simulink model "switching_controller_parallel_after_retraining"  (R2020a)
settings: Solver=FixedStepAuto  StartTime=0.0  StopTime=simulation.time_window  FixedStep=simulation.time_step  MaxStep=.2  RelTol=1e-3
model workspace (MAT data in the model file):
  PID_TRESH = 0.3
undefined symbols (not defined in the file): DiscIntNeverNeededParam
libraries: neural x72, simulink x1
(part 2 of 3)

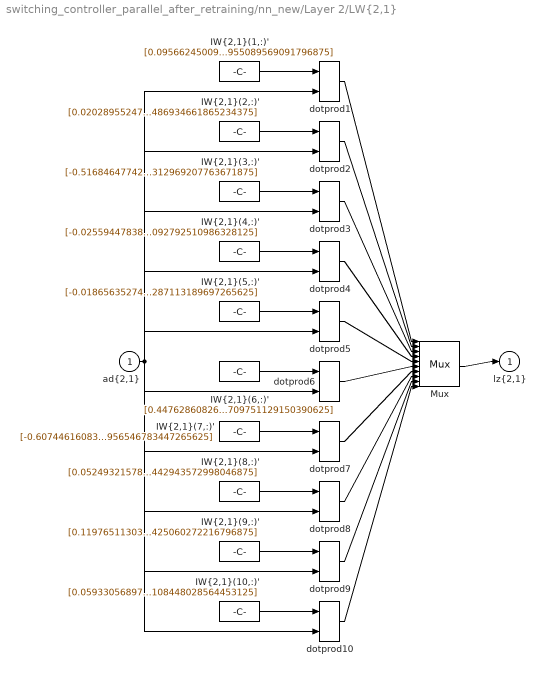
== system switching_controller_parallel_after_retraining/nn_new/Layer 2/LW{2,1} ==
  "ad{2,1}" : Inport  PortDimensions=20
      mask Display: e = 0.06;c1 = [120 230 180]/255;c2 = ([120 230 180]+0)/(256+128);c3 = ([120 230 180]+128)/(256+128);patch([0 1 1 0],[0 0 1 1],c1);patch([0 1 1 1-e 1-e 0+e],[0 0 1 1-e 0+e 0+e],c2);patch([0 0 1 1-e 0+e 0+e],[0 1 1 1-e 1-e 0+e],c3);plot([0 1 1 0 0],[0 0 1 1 0]);
  "IW{2,1}(1,:)'" : Constant  Value=[0.095662450092162620851610199679271318018436431884765625;-0.57681603256735758389339707719045691192150115966796875;0.7629740687628425721555913696647621691226959228515625;0.4894431043993183738649577207979746162891387939453125;0.044507659808209469598505592102810624055564403533935546875;0.61157764582548324039379394889692775905132293701171875;-0.322091177630037084345104858584818430244922637939453125;0.70740757035732826363272351954947225749492645263671875;-0.03743755377230949255018543908590800128877162933349609375;0.6222453992016114820984284961014054715633392333984375;0.307063272338365111924218808781006373465061187744140625;-0.2787568726492377635395314428023993968963623046875;0.059040537912539138576395458812839933671057224273681640625;-0.119200421424518143709292417042888700962066650390625;-0.151215357399669958482490983442403376102447509765625;0.33914961325253145663083387262304313480854034423828125;0.441032178568772248450358119953307323157787322998046875;-0.75715377678111384085468671401031315326690673828125;-0.2200805339957083994750774991189246065914630889892578125;0.54986307386627675253265579158323816955089569091796875]
      mask Display: e = 0.06;c1 = [120 150 230]/255;c2 = ([120 150 230]+0)/383;c3 = ([120 150 230]+128)/383;patch([0 1 1 0],[0 0 1 1],c1);patch([0 1 1 1-e 1-e 0+e],[0 0 1 1-e 0+e 0+e],c2);patch([0 0 1 1-e 0+e 0+e],[0 1 1 1-e 1-e 0+e],c3);plot([0 1 1 0 0],[0 0 1 1 0]);disp('weights');
  "IW{2,1}(10,:)'" : Constant  Value=[0.05933056897562051512640124428799026645720005035400390625;0.2262057047900496165038219942289288155734539031982421875;-0.491182517637794247011839843253255821764469146728515625;0.01215817816725024702595447934072581119835376739501953125;0.375975634012481962908935884115635417401790618896484375;-0.3049767249337567154299222238478250801563262939453125;-0.42157344580778655096509055510978214442729949951171875;-0.2694496021078218728206365994992665946483612060546875;-0.367656953152901255776896505267359316349029541015625;0.274722851495216080497385746639338321983814239501953125;-0.34405620987176710467991824771161191165447235107421875;0.54217418114183357769064741660258732736110687255859375;-0.2419313662361923800148133523180149495601654052734375;-0.044199073428277113606554848956875503063201904296875;0.450309537022767714109505732267280109226703643798828125;-0.2271497176067354961670474722268409095704555511474609375;0.2302888990308247230132110416889190673828125;0.03612319080168803486774464772679493762552738189697265625;-0.45450583955761236776282885330147109925746917724609375;-0.6405685999324095547535762307234108448028564453125]
      mask Display: e = 0.06;c1 = [120 150 230]/255;c2 = ([120 150 230]+0)/383;c3 = ([120 150 230]+128)/383;patch([0 1 1 0],[0 0 1 1],c1);patch([0 1 1 1-e 1-e 0+e],[0 0 1 1-e 0+e 0+e],c2);patch([0 0 1 1-e 0+e 0+e],[0 1 1 1-e 1-e 0+e],c3);plot([0 1 1 0 0],[0 0 1 1 0]);disp('weights');
  "IW{2,1}(2,:)'" : Constant  Value=[0.020289552477637827487821908789555891416966915130615234375;-0.4529280880398627306959724592161364853382110595703125;0.1967778432263952159697595334364450536668300628662109375;-0.422481119070627186840027889047632925212383270263671875;0.360758235334837362717763653563451953232288360595703125;-0.26732116815661643993706775290775112807750701904296875;0.211103401841848115072508562661823816597461700439453125;0.5303785090515169553526675372268073260784149169921875;0.31917976801033953737629644820117391645908355712890625;0.0502309745843228239170485949216526933014392852783203125;-0.1519468024271462269769727981838514097034931182861328125;-0.269186674106762613423171615067985840141773223876953125;-0.13998948573696157193779754379647783935070037841796875;0.0901881135940576783571742680578608997166156768798828125;0.5062996214760033808488515205681324005126953125;-0.472661885555351435339588306305813603103160858154296875;0.413875261618523726525609163218177855014801025390625;0.31956889547999389744603604412986896932125091552734375;0.5147946186520993006041635453584603965282440185546875;0.426550574827694484181250800247653387486934661865234375]
      mask Display: e = 0.06;c1 = [120 150 230]/255;c2 = ([120 150 230]+0)/383;c3 = ([120 150 230]+128)/383;patch([0 1 1 0],[0 0 1 1],c1);patch([0 1 1 1-e 1-e 0+e],[0 0 1 1-e 0+e 0+e],c2);patch([0 0 1 1-e 0+e 0+e],[0 1 1 1-e 1-e 0+e],c3);plot([0 1 1 0 0],[0 0 1 1 0]);disp('weights');
  "IW{2,1}(3,:)'" : Constant  Value=[-0.5168464774227954361407455508015118539333343505859375;-0.1427148876041380576307204819386242888867855072021484375;-0.6662538152277417413671400936436839401721954345703125;-0.0202738475522757123636896636753590428270399570465087890625;0.330811445730504416484762941763619892299175262451171875;-0.04720223712253945880235050935880281031131744384765625;0.47334963592638867879713870934210717678070068359375;0.272869287570113971952423526090569794178009033203125;0.383508624181298440891652035134029574692249298095703125;0.10274607691544514198600523968707420863211154937744140625;-0.48099727776464173967241322316112928092479705810546875;-0.1912774349191261602509683825701358728110790252685546875;-0.48688422303205369789935730295837856829166412353515625;0.2036367915884216006627838169151800684630870819091796875;0.343428109269054981922408842365257441997528076171875;0.34399707401992551947245146948262117803096771240234375;-0.2911771029658838383369356961338780820369720458984375;-0.447043066036233394111576444629463367164134979248046875;0.27467246967589920014773952061659656465053558349609375;-0.17528281692238589783983115921728312969207763671875]
      mask Display: e = 0.06;c1 = [120 150 230]/255;c2 = ([120 150 230]+0)/383;c3 = ([120 150 230]+128)/383;patch([0 1 1 0],[0 0 1 1],c1);patch([0 1 1 1-e 1-e 0+e],[0 0 1 1-e 0+e 0+e],c2);patch([0 0 1 1-e 0+e 0+e],[0 1 1 1-e 1-e 0+e],c3);plot([0 1 1 0 0],[0 0 1 1 0]);disp('weights');
  "IW{2,1}(4,:)'" : Constant  Value=[-0.0255944783879310799878936677487217821180820465087890625;-0.32514893820349699549154820488183759152889251708984375;-0.50495213134970884372165755848982371389865875244140625;-0.08009626728177850207845978047771495766937732696533203125;0.621870632723732885693834759877063333988189697265625;-0.1569360058044794448139924725182936526834964752197265625;0.037051623852388450297556943269228213466703891754150390625;-0.311659061573057172278566895329277031123638153076171875;0.2078238710499483998805914097829372622072696685791015625;0.5261131268857199838606675257324241101741790771484375;-0.02599063693774654459911488402212853543460369110107421875;0.0881885034275140811121929118598927743732929229736328125;-0.56822385294523825027823704658658243715763092041015625;-0.126909132712898886641283979770378209650516510009765625;-0.5497702978723746358724611127399839460849761962890625;-0.1443765114071815236496121315212803892791271209716796875;-0.61709581930341717015409130908665247261524200439453125;-0.2424174009854617450887559471084387041628360748291015625;0.224426304076993876623902224309858866035938262939453125;0.258331430170472220453348199953325092792510986328125]
      mask Display: e = 0.06;c1 = [120 150 230]/255;c2 = ([120 150 230]+0)/383;c3 = ([120 150 230]+128)/383;patch([0 1 1 0],[0 0 1 1],c1);patch([0 1 1 1-e 1-e 0+e],[0 0 1 1-e 0+e 0+e],c2);patch([0 0 1 1-e 0+e 0+e],[0 1 1 1-e 1-e 0+e],c3);plot([0 1 1 0 0],[0 0 1 1 0]);disp('weights');
  "IW{2,1}(5,:)'" : Constant  Value=[-0.018656352749670833401918201843727729283273220062255859375;-0.10100244579175422787731264406829723156988620758056640625;-0.08906911079082380222615711318212561309337615966796875;0.461968780997085215478392683507991023361682891845703125;-0.0641925955297324157822203005707706324756145477294921875;-0.057724015112942062000200849070097319781780242919921875;-0.352857772975186889663490319435368292033672332763671875;-0.52048303324767630773095561380614526569843292236328125;-0.46776209564934212448150674390490166842937469482421875;0.62665385048559729685990760117419995367527008056640625;-0.05359164545710608240636219079533475451171398162841796875;-0.48068861138279361799874322969117201864719390869140625;-0.4300874121532929361677588531165383756160736083984375;0.503059470004075581783808956970460712909698486328125;0.3569004752481521602902603262919001281261444091796875;0.253486227815609754809855758139747194945812225341796875;0.2808896963707583349645346970646642148494720458984375;-0.10195602652315027825125071103684604167938232421875;-0.294562215523830328578469561762176454067230224609375;-0.487670269796994182431859599091694690287113189697265625]
      mask Display: e = 0.06;c1 = [120 150 230]/255;c2 = ([120 150 230]+0)/383;c3 = ([120 150 230]+128)/383;patch([0 1 1 0],[0 0 1 1],c1);patch([0 1 1 1-e 1-e 0+e],[0 0 1 1-e 0+e 0+e],c2);patch([0 0 1 1-e 0+e 0+e],[0 1 1 1-e 1-e 0+e],c3);plot([0 1 1 0 0],[0 0 1 1 0]);disp('weights');
  "IW{2,1}(6,:)'" : Constant  Value=[0.447628608267130079223505845220643095672130584716796875;0.197785098164891370853268881546682678163051605224609375;-0.2408918540521668705256530529368319548666477203369140625;0.410766212020621301892475685235694982111454010009765625;-0.4141113041019461871172779865446500480175018310546875;0.18222575673717766875370216439478099346160888671875;-0.16939486074770082613127897275262512266635894775390625;0.04791024238165515758414159108724561519920825958251953125;1.4184370561259085352645570310414768755435943603515625;-0.42627870064481054868110732058994472026824951171875;0.03013456995836032159541417740911128930747509002685546875;0.0821901968724050302483874475001357495784759521484375;-0.58501686053825296962571655967622064054012298583984375;0.400951383458212406996068466469296254217624664306640625;-0.08461585737425574016423723833213443867862224578857421875;-0.10207911316419748803951961235725320875644683837890625;0.251211721503758200757516760859289206564426422119140625;0.276017713722788382568751330836676061153411865234375;0.55181693210051729892029470647685229778289794921875;-0.23213641069457191523639494334929622709751129150390625]
      mask Display: e = 0.06;c1 = [120 150 230]/255;c2 = ([120 150 230]+0)/383;c3 = ([120 150 230]+128)/383;patch([0 1 1 0],[0 0 1 1],c1);patch([0 1 1 1-e 1-e 0+e],[0 0 1 1-e 0+e 0+e],c2);patch([0 0 1 1-e 0+e 0+e],[0 1 1 1-e 1-e 0+e],c3);plot([0 1 1 0 0],[0 0 1 1 0]);disp('weights');
  "IW{2,1}(7,:)'" : Constant  Value=[-0.60744616083521540961243090350762940943241119384765625;-0.1989567828536343008227760265071992762386798858642578125;-0.1099866679872840424803115411123144440352916717529296875;0.31471386102459930622643469178001396358013153076171875;-0.841768544934840434734724112786352634429931640625;0.257489327361677455829891414396115578711032867431640625;-0.310530242125193256530479857246973551809787750244140625;-0.158849574947457605755829490590258501470088958740234375;-0.338238378029836195270974030790966935455799102783203125;0.788539229652482021037940285168588161468505859375;-0.261832133680638345918367804188164882361888885498046875;-0.68146039698138116680325993002043105661869049072265625;0.312582449672419160346947819562046788632869720458984375;-0.482507481073186583753198419799446128308773040771484375;0.07110183285752659509970641238396638073027133941650390625;-0.17565337853651230570761754279374144971370697021484375;0.162937948573875834856750088874832727015018463134765625;0.7065307135809699712325482323649339377880096435546875;-0.59035250811079753585630669476813636720180511474609375;-0.049137130417979769936298595212065265513956546783447265625]
      mask Display: e = 0.06;c1 = [120 150 230]/255;c2 = ([120 150 230]+0)/383;c3 = ([120 150 230]+128)/383;patch([0 1 1 0],[0 0 1 1],c1);patch([0 1 1 1-e 1-e 0+e],[0 0 1 1-e 0+e 0+e],c2);patch([0 0 1 1-e 0+e 0+e],[0 1 1 1-e 1-e 0+e],c3);plot([0 1 1 0 0],[0 0 1 1 0]);disp('weights');
  "IW{2,1}(8,:)'" : Constant  Value=[0.05249321578110215102963564959281939081847667694091796875;-0.426761081272360343064065091311931610107421875;0.41150645483916736822038728860206902027130126953125;0.127109749863090593091641267164959572255611419677734375;0.38997893629184920971653127708123065531253814697265625;0.380453301748915728719424578230245970189571380615234375;-0.4108039483403225222701848906581290066242218017578125;0.44234762890323919837243238362134434282779693603515625;0.38422075107782249769883264889358542859554290771484375;-0.258439994378828863386132752566481940448284149169921875;-0.038826720633432267038021024063709774054586887359619140625;-0.53476402365100472735548464697785675525665283203125;-0.055864831597369372928607589301464031450450420379638671875;-0.485179454347075544973222349653951823711395263671875;0.1088612177058258245754274184946552850306034088134765625;0.4192271991742699821514861469040624797344207763671875;-0.292194058956679325600447327815345488488674163818359375;0.384120691131496105885645420130458660423755645751953125;-0.419365688597390151581834061289555393159389495849609375;0.052529978561823835458977072221387061290442943572998046875]
      mask Display: e = 0.06;c1 = [120 150 230]/255;c2 = ([120 150 230]+0)/383;c3 = ([120 150 230]+128)/383;patch([0 1 1 0],[0 0 1 1],c1);patch([0 1 1 1-e 1-e 0+e],[0 0 1 1-e 0+e 0+e],c2);patch([0 0 1 1-e 0+e 0+e],[0 1 1 1-e 1-e 0+e],c3);plot([0 1 1 0 0],[0 0 1 1 0]);disp('weights');
  "IW{2,1}(9,:)'" : Constant  Value=[0.11976511303114555084814440988338901661336421966552734375;-0.12117258832265496992786069085923372767865657806396484375;-0.500407631941599095881656467099674046039581298828125;0.07440973515825667627954231875264667905867099761962890625;-0.763806972464987410376124898903071880340576171875;-0.01094096329147310926732661329197071609087288379669189453125;-0.05790294052323001483539854916671174578368663787841796875;-0.04411376321814410028654407369685941375792026519775390625;0.26738860522027152466506549899349920451641082763671875;-0.33300581096538917069693752637249417603015899658203125;-0.483218507813352460278366606871713884174823760986328125;-0.5412747621196107861152313489583320915699005126953125;-0.419437318384453361463926057695061899721622467041015625;-0.45704093626113884152317723419400863349437713623046875;-0.493187989132750581600106443147524259984493255615234375;-0.058655187928478548509136913935435586608946323394775390625;0.0713028538369511466488148698772420175373554229736328125;0.354316933494928487657915638919803313910961151123046875;-0.475823174235289025890693892506533302366733551025390625;0.09016441802686762929663899512888747267425060272216796875]
      mask Display: e = 0.06;c1 = [120 150 230]/255;c2 = ([120 150 230]+0)/383;c3 = ([120 150 230]+128)/383;patch([0 1 1 0],[0 0 1 1],c1);patch([0 1 1 1-e 1-e 0+e],[0 0 1 1-e 0+e 0+e],c2);patch([0 0 1 1-e 0+e 0+e],[0 1 1 1-e 1-e 0+e],c3);plot([0 1 1 0 0],[0 0 1 1 0]);disp('weights');
  Mux : Mux  Inputs=10
      mask Display: e = 0.06;c1 = [120 150 230]/255;c2 = ([120 150 230]+0)/383;c3 = ([120 150 230]+128)/383;patch([0 1 1 0],[0 0 1 1],c1);patch([0 1 1 1-e 1-e 0+e],[0 0 1 1-e 0+e 0+e],c2);patch([0 0 1 1-e 0+e 0+e],[0 1 1 1-e 1-e 0+e],c3);plot([0 1 1 0 0],[0 0 1 1 0]);disp('Mux');
  dotprod{1..10} (10 alike) : neural/Weight Functions/dotprod
  "lz{2,1}" : Outport
      mask Display: e = 0.06;c1 = [120 230 180]/255;c2 = ([120 230 180]+0)/(256+128);c3 = ([120 230 180]+128)/(256+128);patch([0 1 1 0],[0 0 1 1],c1);patch([0 1 1 1-e 1-e 0+e],[0 0 1 1-e 0+e 0+e],c2);patch([0 0 1 1-e 0+e 0+e],[0 1 1 1-e 1-e 0+e],c3);plot([0 1 1 0 0],[0 0 1 1 0]);
  wires:
  "IW{2,1}(1,:)'"/1 -> dotprod1/1
  "ad{2,1}"/1 -> dotprod1/2, dotprod2/2, dotprod3/2, dotprod4/2, dotprod5/2, dotprod6/2, dotprod7/2, dotprod8/2, dotprod9/2, dotprod10/2
  dotprod1/1 -> Mux/1
  "IW{2,1}(2,:)'"/1 -> dotprod2/1
  dotprod2/1 -> Mux/2
  "IW{2,1}(3,:)'"/1 -> dotprod3/1
  dotprod3/1 -> Mux/3
  "IW{2,1}(4,:)'"/1 -> dotprod4/1
  dotprod4/1 -> Mux/4
  "IW{2,1}(5,:)'"/1 -> dotprod5/1
  dotprod5/1 -> Mux/5
  "IW{2,1}(6,:)'"/1 -> dotprod6/1
  dotprod6/1 -> Mux/6
  "IW{2,1}(7,:)'"/1 -> dotprod7/1
  dotprod7/1 -> Mux/7
  "IW{2,1}(8,:)'"/1 -> dotprod8/1
  dotprod8/1 -> Mux/8
  "IW{2,1}(9,:)'"/1 -> dotprod9/1
  dotprod9/1 -> Mux/9
  "IW{2,1}(10,:)'"/1 -> dotprod10/1
  dotprod10/1 -> Mux/10
  Mux/1 -> "lz{2,1}"/1

== system switching_controller_parallel_after_retraining/nn_new/Layer 3/Delays 1 ==
  "p{3}" : Inport  PortDimensions=10
      mask Display: e = 0.06;c1 = [120 230 180]/255;c2 = ([120 230 180]+0)/(256+128);c3 = ([120 230 180]+128)/(256+128);patch([0 1 1 0],[0 0 1 1],c1);patch([0 1 1 1-e 1-e 0+e],[0 0 1 1-e 0+e 0+e],c2);patch([0 0 1 1-e 0+e 0+e],[0 1 1 1-e 1-e 0+e],c3);plot([0 1 1 0 0],[0 0 1 1 0]);
  mux : Mux  Inputs=1
      mask Display: e = 0.06;c1 = [120 150 230]/255;c2 = ([120 150 230]+0)/383;c3 = ([120 150 230]+128)/383;patch([0 1 1 0],[0 0 1 1],c1);patch([0 1 1 1-e 1-e 0+e],[0 0 1 1-e 0+e 0+e],c2);patch([0 0 1 1-e 0+e 0+e],[0 1 1 1-e 1-e 0+e],c3);plot([0 1 1 0 0],[0 0 1 1 0]);disp('Mux')
  "pd{3,2}" : Outport
      mask Display: e = 0.06;c1 = [120 230 180]/255;c2 = ([120 230 180]+0)/(256+128);c3 = ([120 230 180]+128)/(256+128);patch([0 1 1 0],[0 0 1 1],c1);patch([0 1 1 1-e 1-e 0+e],[0 0 1 1-e 0+e 0+e],c2);patch([0 0 1 1-e 0+e 0+e],[0 1 1 1-e 1-e 0+e],c3);plot([0 1 1 0 0],[0 0 1 1 0]);
  wires:
  "p{3}"/1 -> mux/1
  mux/1 -> "pd{3,2}"/1

== system switching_controller_parallel_after_retraining/nn_new/Layer 3/LW{3,2} ==
  "ad{3,2}" : Inport  PortDimensions=10
      mask Display: e = 0.06;c1 = [120 230 180]/255;c2 = ([120 230 180]+0)/(256+128);c3 = ([120 230 180]+128)/(256+128);patch([0 1 1 0],[0 0 1 1],c1);patch([0 1 1 1-e 1-e 0+e],[0 0 1 1-e 0+e 0+e],c2);patch([0 0 1 1-e 0+e 0+e],[0 1 1 1-e 1-e 0+e],c3);plot([0 1 1 0 0],[0 0 1 1 0]);
  "IW{3,2}(1,:)'" : Constant  Value=[1.3105469416649084823944804156781174242496490478515625;0.11434772518992149248351353207908687181770801544189453125;0.141854079167701485619801360371639020740985870361328125;-0.1633213476254641582929849619176820851862430572509765625;-0.1204141857635989409924803794638137333095073699951171875;-0.62874271777680379447161840289481915533542633056640625;0.332205226784654694682785702752880752086639404296875;-0.456611756549471115018690170472837053239345550537109375;0.22544091537273924785722556407563388347625732421875;0.553621473998617386058640477131120860576629638671875]
      mask Display: e = 0.06;c1 = [120 150 230]/255;c2 = ([120 150 230]+0)/383;c3 = ([120 150 230]+128)/383;patch([0 1 1 0],[0 0 1 1],c1);patch([0 1 1 1-e 1-e 0+e],[0 0 1 1-e 0+e 0+e],c2);patch([0 0 1 1-e 0+e 0+e],[0 1 1 1-e 1-e 0+e],c3);plot([0 1 1 0 0],[0 0 1 1 0]);disp('weights');
  Mux : Mux  Inputs=1
      mask Display: e = 0.06;c1 = [120 150 230]/255;c2 = ([120 150 230]+0)/383;c3 = ([120 150 230]+128)/383;patch([0 1 1 0],[0 0 1 1],c1);patch([0 1 1 1-e 1-e 0+e],[0 0 1 1-e 0+e 0+e],c2);patch([0 0 1 1-e 0+e 0+e],[0 1 1 1-e 1-e 0+e],c3);plot([0 1 1 0 0],[0 0 1 1 0]);disp('Mux');
  dotprod1 : neural/Weight Functions/dotprod
  "lz{3,2}" : Outport
      mask Display: e = 0.06;c1 = [120 230 180]/255;c2 = ([120 230 180]+0)/(256+128);c3 = ([120 230 180]+128)/(256+128);patch([0 1 1 0],[0 0 1 1],c1);patch([0 1 1 1-e 1-e 0+e],[0 0 1 1-e 0+e 0+e],c2);patch([0 0 1 1-e 0+e 0+e],[0 1 1 1-e 1-e 0+e],c3);plot([0 1 1 0 0],[0 0 1 1 0]);
  wires:
  "IW{3,2}(1,:)'"/1 -> dotprod1/1
  "ad{3,2}"/1 -> dotprod1/2
  dotprod1/1 -> Mux/1
  Mux/1 -> "lz{3,2}"/1

== system switching_controller_parallel_after_retraining/nn_old/Layer 1/Delays 1 ==
  "p{1}" : Inport  PortDimensions=6
      mask Display: e = 0.06;c1 = [120 230 180]/255;c2 = ([120 230 180]+0)/(256+128);c3 = ([120 230 180]+128)/(256+128);patch([0 1 1 0],[0 0 1 1],c1);patch([0 1 1 1-e 1-e 0+e],[0 0 1 1-e 0+e 0+e],c2);patch([0 0 1 1-e 0+e 0+e],[0 1 1 1-e 1-e 0+e],c3);plot([0 1 1 0 0],[0 0 1 1 0]);
  mux : Mux  Inputs=1
      mask Display: e = 0.06;c1 = [120 150 230]/255;c2 = ([120 150 230]+0)/383;c3 = ([120 150 230]+128)/383;patch([0 1 1 0],[0 0 1 1],c1);patch([0 1 1 1-e 1-e 0+e],[0 0 1 1-e 0+e 0+e],c2);patch([0 0 1 1-e 0+e 0+e],[0 1 1 1-e 1-e 0+e],c3);plot([0 1 1 0 0],[0 0 1 1 0]);disp('Mux')
  "pd{1,1}" : Outport
      mask Display: e = 0.06;c1 = [120 230 180]/255;c2 = ([120 230 180]+0)/(256+128);c3 = ([120 230 180]+128)/(256+128);patch([0 1 1 0],[0 0 1 1],c1);patch([0 1 1 1-e 1-e 0+e],[0 0 1 1-e 0+e 0+e],c2);patch([0 0 1 1-e 0+e 0+e],[0 1 1 1-e 1-e 0+e],c3);plot([0 1 1 0 0],[0 0 1 1 0]);
  wires:
  "p{1}"/1 -> mux/1
  mux/1 -> "pd{1,1}"/1

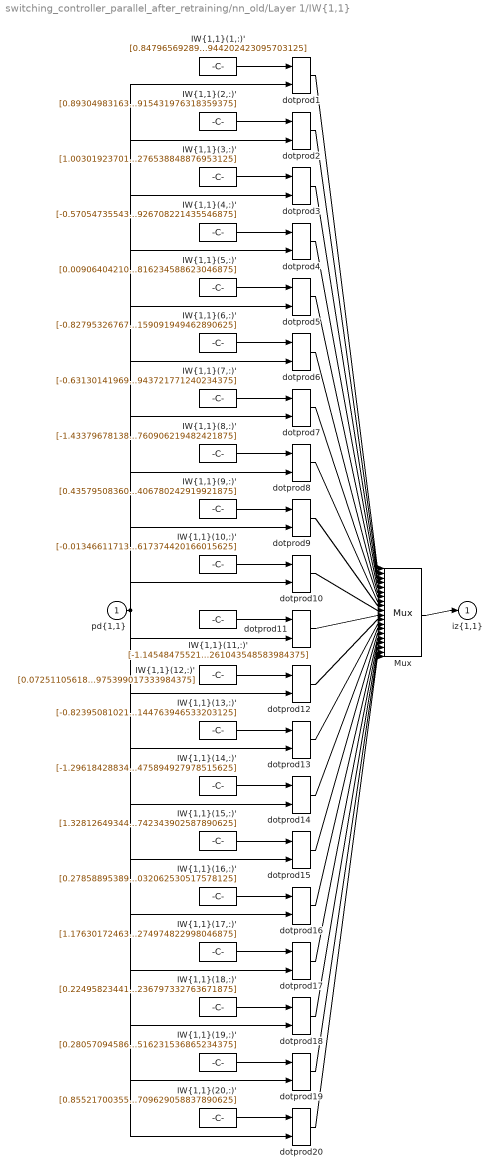
== system switching_controller_parallel_after_retraining/nn_old/Layer 1/IW{1,1} ==
  "pd{1,1}" : Inport  PortDimensions=6
      mask Display: e = 0.06;c1 = [120 230 180]/255;c2 = ([120 230 180]+0)/(256+128);c3 = ([120 230 180]+128)/(256+128);patch([0 1 1 0],[0 0 1 1],c1);patch([0 1 1 1-e 1-e 0+e],[0 0 1 1-e 0+e 0+e],c2);patch([0 0 1 1-e 0+e 0+e],[0 1 1 1-e 1-e 0+e],c3);plot([0 1 1 0 0],[0 0 1 1 0]);
  "IW{1,1}(1,:)'" : Constant  Value=[0.8479656928952004069088843607460148632526397705078125;1.30653730457253569596787201589904725551605224609375;0.4759843172515700882030387219856493175029754638671875;-0.298179296030744944712154165245010517537593841552734375;0.1286761095270509969168415409512817859649658203125;1.1737363862125615998621697144699282944202423095703125]
      mask Display: e = 0.06;c1 = [120 150 230]/255;c2 = ([120 150 230]+0)/383;c3 = ([120 150 230]+128)/383;patch([0 1 1 0],[0 0 1 1],c1);patch([0 1 1 1-e 1-e 0+e],[0 0 1 1-e 0+e 0+e],c2);patch([0 0 1 1-e 0+e 0+e],[0 1 1 1-e 1-e 0+e],c3);plot([0 1 1 0 0],[0 0 1 1 0]);disp('Weights');
  "IW{1,1}(10,:)'" : Constant  Value=[-0.0134661171372473138785341717493793112225830554962158203125;-1.2253406401084934174150475882925093173980712890625;-1.635852065528882182121606092550791800022125244140625;-0.126483801298131248724843089803471229970455169677734375;0.5007659441431915325892987311817705631256103515625;-0.8018994321260122237760015195817686617374420166015625]
      mask Display: e = 0.06;c1 = [120 150 230]/255;c2 = ([120 150 230]+0)/383;c3 = ([120 150 230]+128)/383;patch([0 1 1 0],[0 0 1 1],c1);patch([0 1 1 1-e 1-e 0+e],[0 0 1 1-e 0+e 0+e],c2);patch([0 0 1 1-e 0+e 0+e],[0 1 1 1-e 1-e 0+e],c3);plot([0 1 1 0 0],[0 0 1 1 0]);disp('Weights');
  "IW{1,1}(11,:)'" : Constant  Value=[-1.1454847552134779231636230178992263972759246826171875;0.133993173894402295420746895615593530237674713134765625;1.7605764906283372095430195258813910186290740966796875;1.0367941116706156368110214316402561962604522705078125;0.35828304549271561274537134522688575088977813720703125;-0.313364167699974327518930294900201261043548583984375]
      mask Display: e = 0.06;c1 = [120 150 230]/255;c2 = ([120 150 230]+0)/383;c3 = ([120 150 230]+128)/383;patch([0 1 1 0],[0 0 1 1],c1);patch([0 1 1 1-e 1-e 0+e],[0 0 1 1-e 0+e 0+e],c2);patch([0 0 1 1-e 0+e 0+e],[0 1 1 1-e 1-e 0+e],c3);plot([0 1 1 0 0],[0 0 1 1 0]);disp('Weights');
  "IW{1,1}(12,:)'" : Constant  Value=[0.07251105618688942489047377648603287525475025177001953125;1.40258153356335402150989466463215649127960205078125;-0.2246418606402491580098512713448144495487213134765625;-0.1111410516712949270168309112705173902213573455810546875;-1.6799446626142866545450260673533193767070770263671875;0.73013207717757866443974990033893845975399017333984375]
      mask Display: e = 0.06;c1 = [120 150 230]/255;c2 = ([120 150 230]+0)/383;c3 = ([120 150 230]+128)/383;patch([0 1 1 0],[0 0 1 1],c1);patch([0 1 1 1-e 1-e 0+e],[0 0 1 1-e 0+e 0+e],c2);patch([0 0 1 1-e 0+e 0+e],[0 1 1 1-e 1-e 0+e],c3);plot([0 1 1 0 0],[0 0 1 1 0]);disp('Weights');
  "IW{1,1}(13,:)'" : Constant  Value=[-0.82395081021712923696753705371520482003688812255859375;0.0837908613743596208944808267915504984557628631591796875;0.7709452644446750380069488528533838689327239990234375;0.5053790289739452656903040406177751719951629638671875;1.0473750004361310761424874726799316704273223876953125;-1.8529480789745929047995787186664529144763946533203125]
      mask Display: e = 0.06;c1 = [120 150 230]/255;c2 = ([120 150 230]+0)/383;c3 = ([120 150 230]+128)/383;patch([0 1 1 0],[0 0 1 1],c1);patch([0 1 1 1-e 1-e 0+e],[0 0 1 1-e 0+e 0+e],c2);patch([0 0 1 1-e 0+e 0+e],[0 1 1 1-e 1-e 0+e],c3);plot([0 1 1 0 0],[0 0 1 1 0]);disp('Weights');
  "IW{1,1}(14,:)'" : Constant  Value=[-1.296184288346896806842778460122644901275634765625;0.9147936201889892426919459467171691358089447021484375;-0.9618052347369945298538596034632064402103424072265625;-0.039133632145276438241143779350750264711678028106689453125;0.509195428205596822834877457353286445140838623046875;0.98351998404680485155182623202563263475894927978515625]
      mask Display: e = 0.06;c1 = [120 150 230]/255;c2 = ([120 150 230]+0)/383;c3 = ([120 150 230]+128)/383;patch([0 1 1 0],[0 0 1 1],c1);patch([0 1 1 1-e 1-e 0+e],[0 0 1 1-e 0+e 0+e],c2);patch([0 0 1 1-e 0+e 0+e],[0 1 1 1-e 1-e 0+e],c3);plot([0 1 1 0 0],[0 0 1 1 0]);disp('Weights');
  "IW{1,1}(15,:)'" : Constant  Value=[1.328126493443487987633488955907523632049560546875;0.73966379721295627547306139604188501834869384765625;-0.047092984815939591125566465734664234332740306854248046875;-1.532780146204789417652136762626469135284423828125;0.5872130739696117540660225131432525813579559326171875;-0.2055319285752058855454293961884104646742343902587890625]
      mask Display: e = 0.06;c1 = [120 150 230]/255;c2 = ([120 150 230]+0)/383;c3 = ([120 150 230]+128)/383;patch([0 1 1 0],[0 0 1 1],c1);patch([0 1 1 1-e 1-e 0+e],[0 0 1 1-e 0+e 0+e],c2);patch([0 0 1 1-e 0+e 0+e],[0 1 1 1-e 1-e 0+e],c3);plot([0 1 1 0 0],[0 0 1 1 0]);disp('Weights');
  "IW{1,1}(16,:)'" : Constant  Value=[0.278588953897926983049870841568917967379093170166015625;0.24722436134048952904862517243600450456142425537109375;0.4999783272710069947919464539154432713985443115234375;-0.2260918572217274213898008383694104850292205810546875;-1.8108150464917540656273331478587351739406585693359375;1.53811760352148940711458635632880032062530517578125]
      mask Display: e = 0.06;c1 = [120 150 230]/255;c2 = ([120 150 230]+0)/383;c3 = ([120 150 230]+128)/383;patch([0 1 1 0],[0 0 1 1],c1);patch([0 1 1 1-e 1-e 0+e],[0 0 1 1-e 0+e 0+e],c2);patch([0 0 1 1-e 0+e 0+e],[0 1 1 1-e 1-e 0+e],c3);plot([0 1 1 0 0],[0 0 1 1 0]);disp('Weights');
  "IW{1,1}(17,:)'" : Constant  Value=[1.17630172463046189790247808559797704219818115234375;-0.64719651203503525405125174074782989919185638427734375;-0.95661663581220268692817398914485238492488861083984375;1.227169923518439897947018835111521184444427490234375;0.84879784929610024857282724042306654155254364013671875;-0.74668647718154967929393706072005443274974822998046875]
      mask Display: e = 0.06;c1 = [120 150 230]/255;c2 = ([120 150 230]+0)/383;c3 = ([120 150 230]+128)/383;patch([0 1 1 0],[0 0 1 1],c1);patch([0 1 1 1-e 1-e 0+e],[0 0 1 1-e 0+e 0+e],c2);patch([0 0 1 1-e 0+e 0+e],[0 1 1 1-e 1-e 0+e],c3);plot([0 1 1 0 0],[0 0 1 1 0]);disp('Weights');
  "IW{1,1}(18,:)'" : Constant  Value=[0.22495823441322093660943437498644925653934478759765625;0.16280166849995814093432500158087350428104400634765625;0.054426777374156097566437750856493948958814144134521484375;1.5190168114950932665152549816411919891834259033203125;1.202302949988925728774802337284199893474578857421875;-0.63654376405440415975789392177830450236797332763671875]
      mask Display: e = 0.06;c1 = [120 150 230]/255;c2 = ([120 150 230]+0)/383;c3 = ([120 150 230]+128)/383;patch([0 1 1 0],[0 0 1 1],c1);patch([0 1 1 1-e 1-e 0+e],[0 0 1 1-e 0+e 0+e],c2);patch([0 0 1 1-e 0+e 0+e],[0 1 1 1-e 1-e 0+e],c3);plot([0 1 1 0 0],[0 0 1 1 0]);disp('Weights');
  "IW{1,1}(19,:)'" : Constant  Value=[0.28057094586534725433324410914792679250240325927734375;-1.1316660455487894676451787745463661849498748779296875;-0.31985145050699514968073344789445400238037109375;-0.7046752862369860537228305474855005741119384765625;1.253498611021385489294743820209987461566925048828125;-1.2499253664823848364306968505843542516231536865234375]
      mask Display: e = 0.06;c1 = [120 150 230]/255;c2 = ([120 150 230]+0)/383;c3 = ([120 150 230]+128)/383;patch([0 1 1 0],[0 0 1 1],c1);patch([0 1 1 1-e 1-e 0+e],[0 0 1 1-e 0+e 0+e],c2);patch([0 0 1 1-e 0+e 0+e],[0 1 1 1-e 1-e 0+e],c3);plot([0 1 1 0 0],[0 0 1 1 0]);disp('Weights');
  "IW{1,1}(2,:)'" : Constant  Value=[0.8930498316379973378076329026953317224979400634765625;1.5759542690744046122830468448228202760219573974609375;0.69741571313243999608033618642366491258144378662109375;-0.9848192024209374562104812866891734302043914794921875;0.591042629404637143153422584873624145984649658203125;0.1806729757254300350322040458195260725915431976318359375]
      mask Display: e = 0.06;c1 = [120 150 230]/255;c2 = ([120 150 230]+0)/383;c3 = ([120 150 230]+128)/383;patch([0 1 1 0],[0 0 1 1],c1);patch([0 1 1 1-e 1-e 0+e],[0 0 1 1-e 0+e 0+e],c2);patch([0 0 1 1-e 0+e 0+e],[0 1 1 1-e 1-e 0+e],c3);plot([0 1 1 0 0],[0 0 1 1 0]);disp('Weights');
  "IW{1,1}(20,:)'" : Constant  Value=[0.85521700355193031040101914186379872262477874755859375;0.4053140014737433016733803015085868537425994873046875;-1.187054090459810584690103496541269123554229736328125;-0.71263434180851203958440009955666027963161468505859375;1.186819031215439412818568598595447838306427001953125;-0.82403958168427815511591916219913400709629058837890625]
      mask Display: e = 0.06;c1 = [120 150 230]/255;c2 = ([120 150 230]+0)/383;c3 = ([120 150 230]+128)/383;patch([0 1 1 0],[0 0 1 1],c1);patch([0 1 1 1-e 1-e 0+e],[0 0 1 1-e 0+e 0+e],c2);patch([0 0 1 1-e 0+e 0+e],[0 1 1 1-e 1-e 0+e],c3);plot([0 1 1 0 0],[0 0 1 1 0]);disp('Weights');
  "IW{1,1}(3,:)'" : Constant  Value=[1.00301923701714112979743731557391583919525146484375;-1.2645102014022795433589863023371435701847076416015625;0.9235457146307906040050283991149626672267913818359375;-1.2410789654570664186650219562579877674579620361328125;-0.24137998456902287625069902787799946963787078857421875;-0.77284505193702390801746560100582428276538848876953125]
      mask Display: e = 0.06;c1 = [120 150 230]/255;c2 = ([120 150 230]+0)/383;c3 = ([120 150 230]+128)/383;patch([0 1 1 0],[0 0 1 1],c1);patch([0 1 1 1-e 1-e 0+e],[0 0 1 1-e 0+e 0+e],c2);patch([0 0 1 1-e 0+e 0+e],[0 1 1 1-e 1-e 0+e],c3);plot([0 1 1 0 0],[0 0 1 1 0]);disp('Weights');
  "IW{1,1}(4,:)'" : Constant  Value=[-0.57054735543445700418629940031678415834903717041015625;1.0985124078277508363754577658255584537982940673828125;1.4328136378936349171198116891901008784770965576171875;-0.94042083043369883998963132398785091936588287353515625;-0.83631556734155465537838836098671890795230865478515625;-0.155547418012604576897928154721739701926708221435546875]
      mask Display: e = 0.06;c1 = [120 150 230]/255;c2 = ([120 150 230]+0)/383;c3 = ([120 150 230]+128)/383;patch([0 1 1 0],[0 0 1 1],c1);patch([0 1 1 1-e 1-e 0+e],[0 0 1 1-e 0+e 0+e],c2);patch([0 0 1 1-e 0+e 0+e],[0 1 1 1-e 1-e 0+e],c3);plot([0 1 1 0 0],[0 0 1 1 0]);disp('Weights');
  "IW{1,1}(5,:)'" : Constant  Value=[0.009064042101917003935174221851411857642233371734619140625;0.222282644749310254184138102573342621326446533203125;0.6028400101315483095021363624255172908306121826171875;-1.6130090755166619498339741767267696559429168701171875;1.4038383740851594350118602960719726979732513427734375;-1.21539236116889792782558288308791816234588623046875]
      mask Display: e = 0.06;c1 = [120 150 230]/255;c2 = ([120 150 230]+0)/383;c3 = ([120 150 230]+128)/383;patch([0 1 1 0],[0 0 1 1],c1);patch([0 1 1 1-e 1-e 0+e],[0 0 1 1-e 0+e 0+e],c2);patch([0 0 1 1-e 0+e 0+e],[0 1 1 1-e 1-e 0+e],c3);plot([0 1 1 0 0],[0 0 1 1 0]);disp('Weights');
  "IW{1,1}(6,:)'" : Constant  Value=[-0.8279532676701533144836275823763571679592132568359375;1.267069828731218539275005241506733000278472900390625;0.1580631965590118814812825576154864393174648284912109375;-0.594657404289065549818360523204319179058074951171875;-0.89674220291302442209513401394360698759555816650390625;-1.1159839746367092860879211002611555159091949462890625]
      mask Display: e = 0.06;c1 = [120 150 230]/255;c2 = ([120 150 230]+0)/383;c3 = ([120 150 230]+128)/383;patch([0 1 1 0],[0 0 1 1],c1);patch([0 1 1 1-e 1-e 0+e],[0 0 1 1-e 0+e 0+e],c2);patch([0 0 1 1-e 0+e 0+e],[0 1 1 1-e 1-e 0+e],c3);plot([0 1 1 0 0],[0 0 1 1 0]);disp('Weights');
  "IW{1,1}(7,:)'" : Constant  Value=[-0.6313014196923878440514954490936361253261566162109375;0.09103878365153199314629972604961949400603771209716796875;0.38399827792243124147120170164271257817745208740234375;-2.38191775228679336606774086249060928821563720703125;-0.35212675147842975587053615527111105620861053466796875;2.271360282133880303945261402986943721771240234375]
      mask Display: e = 0.06;c1 = [120 150 230]/255;c2 = ([120 150 230]+0)/383;c3 = ([120 150 230]+128)/383;patch([0 1 1 0],[0 0 1 1],c1);patch([0 1 1 1-e 1-e 0+e],[0 0 1 1-e 0+e 0+e],c2);patch([0 0 1 1-e 0+e 0+e],[0 1 1 1-e 1-e 0+e],c3);plot([0 1 1 0 0],[0 0 1 1 0]);disp('Weights');
  "IW{1,1}(8,:)'" : Constant  Value=[-1.4337967813888086165974300456582568585872650146484375;-0.048887678448340098069646586509406915865838527679443359375;0.387358756251124980440891931721125729382038116455078125;0.98598144418065880589807647993438877165317535400390625;-1.2039171562222741318493035578285343945026397705078125;-0.465277755653387081746785725044901482760906219482421875]
      mask Display: e = 0.06;c1 = [120 150 230]/255;c2 = ([120 150 230]+0)/383;c3 = ([120 150 230]+128)/383;patch([0 1 1 0],[0 0 1 1],c1);patch([0 1 1 1-e 1-e 0+e],[0 0 1 1-e 0+e 0+e],c2);patch([0 0 1 1-e 0+e 0+e],[0 1 1 1-e 1-e 0+e],c3);plot([0 1 1 0 0],[0 0 1 1 0]);disp('Weights');
  "IW{1,1}(9,:)'" : Constant  Value=[0.435795083609810729452505029257736168801784515380859375;0.669713991519877982483421874349005520343780517578125;-1.5416725315515587002579422915005125105381011962890625;-0.387866277192614072877319131293916143476963043212890625;-0.53614317691681190325425632181577384471893310546875;-0.3655182822947018461690049662138335406780242919921875]
      mask Display: e = 0.06;c1 = [120 150 230]/255;c2 = ([120 150 230]+0)/383;c3 = ([120 150 230]+128)/383;patch([0 1 1 0],[0 0 1 1],c1);patch([0 1 1 1-e 1-e 0+e],[0 0 1 1-e 0+e 0+e],c2);patch([0 0 1 1-e 0+e 0+e],[0 1 1 1-e 1-e 0+e],c3);plot([0 1 1 0 0],[0 0 1 1 0]);disp('Weights');
  Mux : Mux  Inputs=20
      mask Display: e = 0.06;c1 = [120 150 230]/255;c2 = ([120 150 230]+0)/383;c3 = ([120 150 230]+128)/383;patch([0 1 1 0],[0 0 1 1],c1);patch([0 1 1 1-e 1-e 0+e],[0 0 1 1-e 0+e 0+e],c2);patch([0 0 1 1-e 0+e 0+e],[0 1 1 1-e 1-e 0+e],c3);plot([0 1 1 0 0],[0 0 1 1 0]);disp('Mux');
  dotprod{1..20} (20 alike) : neural/Weight Functions/dotprod
  "iz{1,1}" : Outport
      mask Display: e = 0.06;c1 = [120 230 180]/255;c2 = ([120 230 180]+0)/(256+128);c3 = ([120 230 180]+128)/(256+128);patch([0 1 1 0],[0 0 1 1],c1);patch([0 1 1 1-e 1-e 0+e],[0 0 1 1-e 0+e 0+e],c2);patch([0 0 1 1-e 0+e 0+e],[0 1 1 1-e 1-e 0+e],c3);plot([0 1 1 0 0],[0 0 1 1 0]);
  wires:
  "IW{1,1}(1,:)'"/1 -> dotprod1/1
  "pd{1,1}"/1 -> dotprod1/2, dotprod2/2, dotprod3/2, dotprod4/2, dotprod5/2, dotprod6/2, dotprod7/2, dotprod8/2, dotprod9/2, dotprod10/2, dotprod11/2, dotprod12/2, dotprod13/2, dotprod14/2, dotprod15/2, dotprod16/2, dotprod17/2, dotprod18/2, dotprod19/2, dotprod20/2
  dotprod1/1 -> Mux/1
  "IW{1,1}(2,:)'"/1 -> dotprod2/1
  dotprod2/1 -> Mux/2
  "IW{1,1}(3,:)'"/1 -> dotprod3/1
  dotprod3/1 -> Mux/3
  "IW{1,1}(4,:)'"/1 -> dotprod4/1
  dotprod4/1 -> Mux/4
  "IW{1,1}(5,:)'"/1 -> dotprod5/1
  dotprod5/1 -> Mux/5
  "IW{1,1}(6,:)'"/1 -> dotprod6/1
  dotprod6/1 -> Mux/6
  "IW{1,1}(7,:)'"/1 -> dotprod7/1
  dotprod7/1 -> Mux/7
  "IW{1,1}(8,:)'"/1 -> dotprod8/1
  dotprod8/1 -> Mux/8
  "IW{1,1}(9,:)'"/1 -> dotprod9/1
  dotprod9/1 -> Mux/9
  "IW{1,1}(10,:)'"/1 -> dotprod10/1
  dotprod10/1 -> Mux/10
  "IW{1,1}(11,:)'"/1 -> dotprod11/1
  dotprod11/1 -> Mux/11
  "IW{1,1}(12,:)'"/1 -> dotprod12/1
  dotprod12/1 -> Mux/12
  "IW{1,1}(13,:)'"/1 -> dotprod13/1
  dotprod13/1 -> Mux/13
  "IW{1,1}(14,:)'"/1 -> dotprod14/1
  dotprod14/1 -> Mux/14
  "IW{1,1}(15,:)'"/1 -> dotprod15/1
  dotprod15/1 -> Mux/15
  "IW{1,1}(16,:)'"/1 -> dotprod16/1
  dotprod16/1 -> Mux/16
  "IW{1,1}(17,:)'"/1 -> dotprod17/1
  dotprod17/1 -> Mux/17
  "IW{1,1}(18,:)'"/1 -> dotprod18/1
  dotprod18/1 -> Mux/18
  "IW{1,1}(19,:)'"/1 -> dotprod19/1
  dotprod19/1 -> Mux/19
  "IW{1,1}(20,:)'"/1 -> dotprod20/1
  dotprod20/1 -> Mux/20
  Mux/1 -> "iz{1,1}"/1

== system switching_controller_parallel_after_retraining/nn_old/Layer 2/Delays 1 ==
  "p{2}" : Inport  PortDimensions=20
      mask Display: e = 0.06;c1 = [120 230 180]/255;c2 = ([120 230 180]+0)/(256+128);c3 = ([120 230 180]+128)/(256+128);patch([0 1 1 0],[0 0 1 1],c1);patch([0 1 1 1-e 1-e 0+e],[0 0 1 1-e 0+e 0+e],c2);patch([0 0 1 1-e 0+e 0+e],[0 1 1 1-e 1-e 0+e],c3);plot([0 1 1 0 0],[0 0 1 1 0]);
  mux : Mux  Inputs=1
      mask Display: e = 0.06;c1 = [120 150 230]/255;c2 = ([120 150 230]+0)/383;c3 = ([120 150 230]+128)/383;patch([0 1 1 0],[0 0 1 1],c1);patch([0 1 1 1-e 1-e 0+e],[0 0 1 1-e 0+e 0+e],c2);patch([0 0 1 1-e 0+e 0+e],[0 1 1 1-e 1-e 0+e],c3);plot([0 1 1 0 0],[0 0 1 1 0]);disp('Mux')
  "pd{2,1}" : Outport
      mask Display: e = 0.06;c1 = [120 230 180]/255;c2 = ([120 230 180]+0)/(256+128);c3 = ([120 230 180]+128)/(256+128);patch([0 1 1 0],[0 0 1 1],c1);patch([0 1 1 1-e 1-e 0+e],[0 0 1 1-e 0+e 0+e],c2);patch([0 0 1 1-e 0+e 0+e],[0 1 1 1-e 1-e 0+e],c3);plot([0 1 1 0 0],[0 0 1 1 0]);
  wires:
  "p{2}"/1 -> mux/1
  mux/1 -> "pd{2,1}"/1
